simulink model "speedcontrol1phIM"  (R2023a)
settings: Solver=VariableStepAuto  StartTime=0.0  StopTime=10.0  RelTol=1e-3
undefined symbols (not defined in the file): Capacitor, DiscIntNeverNeededParam, Run, Start
libraries: spsIGBTDiodeLib x4, simulink x2, spsDCVoltageSourceLib x1, spsSinglePhaseAsynchronousMachineLib x1, sps_lib x1
settings Model: Creator=Sandesh  LastModifiedBy=Sandesh

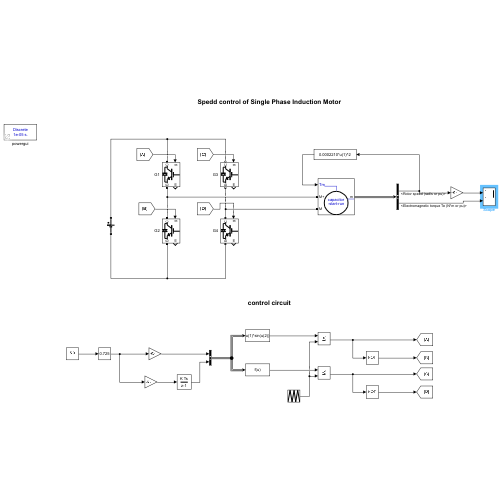
[thumbnail: Simulink's stored preview of the top-level diagram]
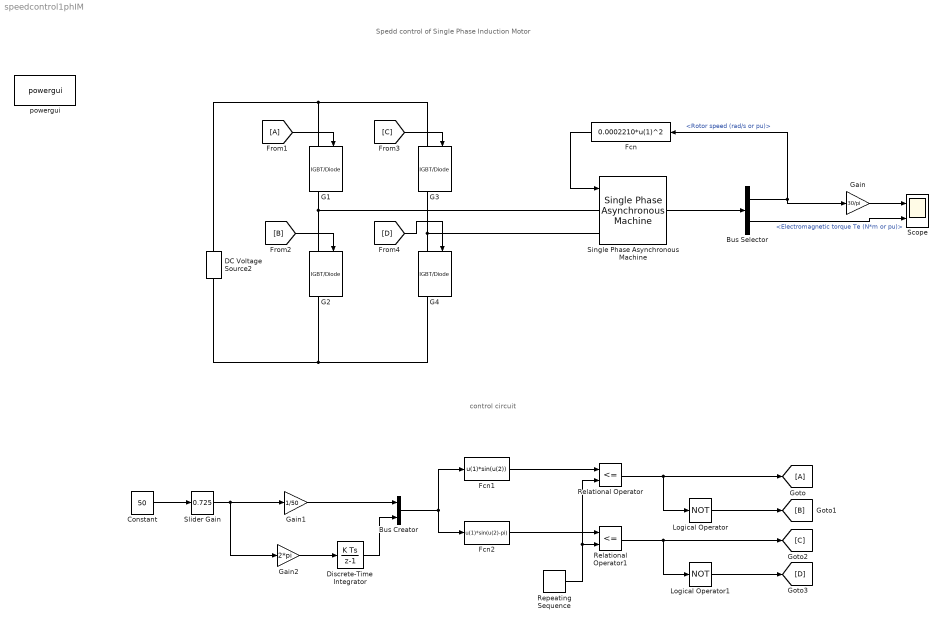
== system speedcontrol1phIM ==
  note: Spedd control of Single Phase Induction Motor
  note: control circuit
  Bus Creator : BusCreator  Inputs=2
  Bus Selector : BusSelector  OutputSignals=Mechanical.Rotor speed (rad/s or pu),Mechanical.Electromagnetic torque Te (N*m or pu)
  Constant : Constant  Value=50
  DC Voltage Source2 : spsDCVoltageSourceLib/DC Voltage Source  Amplitude=100  Measurements=None
  Discrete-Time Integrator : DiscreteIntegrator  SampleTime=-1  ICPrevOutput=DiscIntNeverNeededParam  ICPrevScaledInput=DiscIntNeverNeededParam
  Fcn : Fcn  Expr=0.0002210*u(1)^2
  Fcn1 : Fcn  Expr=u(1)*sin(u(2))
  Fcn2 : Fcn  Expr=u(1)*sin(u(2)-pi)
  From1 : From
  G{1..4} (4 alike) : spsIGBTDiodeLib/IGBT//Diode  Ron=1e-3  Rs=1e5  Cs=inf  Measurements=on
  Gain : Gain  Gain=30/pi
  Gain1 : Gain  Gain=1/50
  Gain2 : Gain  Gain=2*pi
  Goto : Goto
  Logical Operator : Logic  Operator=NOT  AllPortsSameDT=off  OutDataTypeStr=boolean
  Logical Operator1 : Logic  Operator=NOT  AllPortsSameDT=off  OutDataTypeStr=boolean
  Relational Operator : RelationalOperator  Operator=<=  OutDataTypeStr=boolean  RndMeth=Simplest  InputSameDT=off
  Relational Operator1 : RelationalOperator  Operator=<=  OutDataTypeStr=boolean  RndMeth=Simplest  InputSameDT=off
  Repeating Sequence : simulink/Sources/Repeating Sequence  rep_seq_t=[0 1 2]*(1/5000)  rep_seq_y=[-1 1 -1]
  Scope : Scope  NumInputPorts=2
  Single Phase Asynchronous Machine : spsSinglePhaseAsynchronousMachineLib/Single Phase Asynchronous Machine  MechanicalLoad=Torque Tm  UNITS=SI  MachineType=Capacitor-Start-Run  MeasurementBus=off  NominalParameters="[ 746  230  50]"  MainWindingStator="[2.02  7.4e-3]"  MainWindingRotor="[4.12  5.6e-3]"  MutualInductance=0.1772  AuxiliaryWinding="[7.14  8.5e-3]"  Mechanical="[0.0146  0  2 1.18]"  CapacitorStart="[2  254.7e-6]"  CapacitorRun="[18  21.1e-6]"  DisconnectionSpeed=75  InitialSpeed=0  DataType=SI  TsPowergui=0  TsBlock=-1
      settings: LibrarySourceBlock=|
      | sps_lib/Electrical Machines/Single Phase
      | Asynchronous Machine
  Slider Gain : simulink/Math Operations/Slider Gain  gain=0.725  low=.5  high=2
  powergui : sps_lib/powergui  Priority=1  SimulationMode=Discrete  SampleTime=1e-5  frequency=60  Iterations=50  frequencyindice=50  Pbase=100e6  ErrMax=1e-4  UnitsV=kV  UnitsW=MW  buscounter=0  FunctionMessages=off  echomessages=off  EnableUseOfTLC=off  CurrentSourceSwitches=off  DisableSnubberDevices=off  DisableRonSwitches=off  DisableVfSwitches=off  DisplayEquations=off  AutomaticDiscreteSolvers=off  SolverType=Tustin/Backward Euler (TBE)  Interpol=off  ExternalGateDelay=off  methode=off  Ts=100  x0status=blocks  SPID=on  SwTol=0  HookPort=off  NonlinearTolerance=1e-4  nMaxIteration=100  ContinueOnMaxIteration=off  RestoreLinks=warning  ResistiveCurrentMeasurement=off  Frange=[0:2:500]  Ylog=off  Xlog=on  ShowGrid=off  save=off  variable=ZData  structure=0  ZoomFFT=off  StartTime=0.0  cycles=1  DisplayStyle=1  fundamental=60  FreqAxis=off  MaxFrequency=1000  frequencyindicesteady=1  RmsSteady=1  display=off
  wires:
  Single Phase Asynchronous Machine/1 -> Bus Selector/1
  Bus Selector/1 -> Fcn/1, Gain/1  "<Rotor speed (rad/s or pu)>"
  Gain/1 -> Scope/1
  Bus Selector/2 -> Scope/2  "<Electromagnetic torque Te (N*m or pu)>"
  Fcn/1 -> Single Phase Asynchronous Machine/1
  Gain2/1 -> Discrete-Time Integrator/1
  Gain1/1 -> Bus Creator/1
  Discrete-Time Integrator/1 -> Bus Creator/2
  Bus Creator/1 -> Fcn2/1, Fcn1/1
  Fcn1/1 -> Relational Operator/1
  Fcn2/1 -> Relational Operator1/1
  Repeating Sequence/1 -> Relational Operator/2, Relational Operator1/2
  Relational Operator/1 -> Logical Operator/1, Goto/1
  Logical Operator/1 -> [B]
  Relational Operator1/1 -> Logical Operator1/1, [C]
  Logical Operator1/1 -> [D]
  From1/1 -> G1/1
  [B] -> G2/1
  [C] -> G3/1
  [D] -> G4/1
  Constant/1 -> Slider Gain/1
  Slider Gain/1 -> Gain2/1, Gain1/1
  connections:
  G2/LConn1 -- Single Phase Asynchronous Machine/LConn1 -- G1/RConn1
  G4/LConn1 -- Single Phase Asynchronous Machine/LConn2 -- G3/RConn1
  DC Voltage Source2/RConn1 -- G1/LConn1 -- G3/LConn1
  DC Voltage Source2/LConn1 -- G2/RConn1 -- G4/RConn1
